simulink model "Electric_Vehicle_Dynamic"  (R2019a)
settings: Solver=VariableStepAuto  StartTime=0.0  StopTime=10.0  RelTol=1e-3
settings Model: Creator=dağlar  LastModifiedBy=dağlar

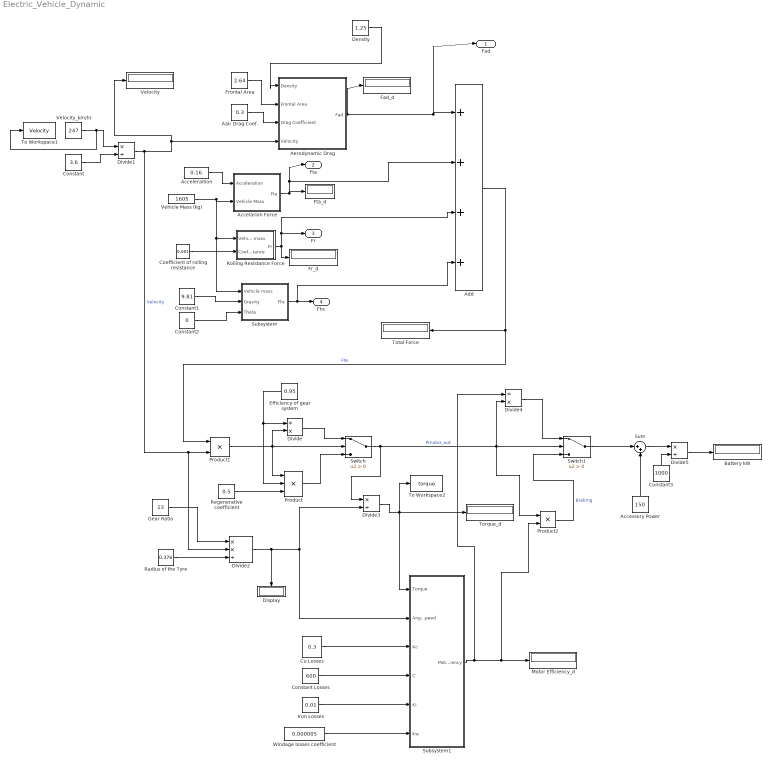
== system Electric_Vehicle_Dynamic ==
  Aair Drag Coef. : Constant  Value=0.3
  Accelarion Force : Subsystem
  Acceleraition : Constant  Value=0.16
  Accessory Power : Constant  Value=150
  Add : Sum  Inputs=++++
  "Aerodynamic Drag " : Subsystem
  Battery kW : Display
  Coefficient of rolling resistance : Constant  Value=0.001
  Constant : Constant  Value=3.6
  Constant Losses : Constant  Value=600
  Constant1 : Constant  Value=9.81
  Constant2 : Constant  Value=0
  Constant3 : Constant  Value=1000
  Cu Losses : Constant  Value=0.3
  Density : Constant  Value=1.25
  Display : Display
  Divide : Product  Inputs=/*
  Divide1 : Product  Inputs=*/
  Divide2 : Product  Inputs=**/
  Divide3 : Product  Inputs=*/
  Divide4 : Product  Inputs=/*
  Divide5 : Product  Inputs=*/
  Efficiency of gear system : Constant  Value=0.95
  "Fad_d " : Display
  Fr_d : Display
  Frontal Area : Constant  Value=2.64
  Fta_d : Display
  Gear Ratio : Constant  Value=13
  Iron Losses : Constant  Value=0.01
  Motor Efficiency_d : Display
  Product : Product  Inputs=3
  Product1 : Product
  Product2 : Product
  Radius of the Tyre : Constant  Value=0.376
  Regenerative coefficient : Constant  Value=0.5
  Rolling Resistance Force : Subsystem
  Subsystem : Subsystem
  Subsystem1 : Subsystem
  Sum : Sum  Inputs=|++
  Switch : Switch  Criteria=u2 > Threshold
  Switch1 : Switch  Criteria=u2 > Threshold
  To Workspace1 : ToWorkspace  VariableName=Velocity  SaveFormat=Timeseries  SampleTime=-1
  To Workspace2 : ToWorkspace  VariableName=torque  SaveFormat=Timeseries  SampleTime=-1
  Torque_d : Display
  Total Force : Display
  Vehicle Mass (kg) : Constant  Value=1605
  Velocity : Display
  Velocity_km/hr : Constant  Value=247
  Windage losses coefficient : Constant  Value=0.000005
  Fad : Outport
  Fta : Outport  Port=2
  Fr : Outport  Port=3
  Fhc : Outport  Port=4
  wires:
  Regenerative coefficient/1 -> Product/3
  Divide/1 -> Switch/1
  Product/1 -> Switch/3
  Efficiency of gear system/1 -> Product/2, Divide/1
  Density/1 -> "Aerodynamic Drag "/1(Density)
  Frontal Area/1 -> "Aerodynamic Drag "/2(Frontal Area)
  Aair Drag Coef./1 -> "Aerodynamic Drag "/3(Drag Coefficient)
  "Aerodynamic Drag "/1(Fad) -> Add/1, Fad/1, "Fad_d "/1
  Velocity_km/hr/1 -> To Workspace1/1, Divide1/1
  Constant/1 -> Divide1/2
  Divide1/1 -> Divide2/2, Product1/2, "Aerodynamic Drag "/4(Velocity), Velocity/1  "Velocity"
  Acceleraition/1 -> Accelarion Force/1(Acceleration)
  Vehicle Mass (kg)/1 -> Accelarion Force/2(Vehicle Mass), Rolling Resistance Force/1(Vehicle mass), Subsystem/1(Vehicle mass)
  Accelarion Force/1(Fta) -> Add/2, Fta/1, Fta_d/1
  Coefficient of rolling resistance/1 -> Rolling Resistance Force/2(Coefficient of rolling resistance)
  Rolling Resistance Force/1(Fr) -> Fr_d/1, Add/3, Fr/1
  Constant1/1 -> Subsystem/2(Gravity)
  Subsystem/1(Fhc) -> Add/4, Fhc/1
  Constant2/1 -> Subsystem/3(Theta)
  Add/1 -> Total Force/1, Product1/1  "Fte"
  Product1/1 -> Divide/2, Product/1, Switch/2
  Gear Ratio/1 -> Divide2/1
  Radius of the Tyre/1 -> Divide2/3
  Divide2/1 -> Display/1, Subsystem1/2(Angular Speed), Divide3/2
  Switch/1 -> Product2/1, Switch1/2, Divide4/2, Divide3/1  "Pmotor_out"
  Divide3/1 -> Torque_d/1, Subsystem1/1("Torque "), To Workspace2/1
  Divide4/1 -> Switch1/1
  Subsystem1/1(Motor Efficiency) -> Divide4/1, Product2/2, Motor Efficiency_d/1
  Cu Losses/1 -> Subsystem1/3(Kc)
  Constant Losses/1 -> Subsystem1/4(C)
  Product2/1 -> Switch1/3  "Braking"
  Switch1/1 -> Sum/1
  Accessory Power/1 -> Sum/2
  Iron Losses/1 -> Subsystem1/5(Ki)
  Windage losses coefficient/1 -> Subsystem1/6(Kw)
  Sum/1 -> Divide5/1
  Constant3/1 -> Divide5/2
  Divide5/1 -> Battery kW/1

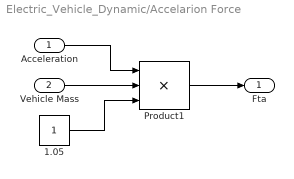
== system Electric_Vehicle_Dynamic/Accelarion Force ==
  Acceleration : Inport
  Vehicle Mass : Inport  Port=2
  "1.05 " : Constant
  Product1 : Product  Inputs=3
  Fta : Outport
  wires:
  "1.05 "/1 -> Product1/3
  Vehicle Mass/1 -> Product1/2
  Product1/1 -> Fta/1
  Acceleration/1 -> Product1/1

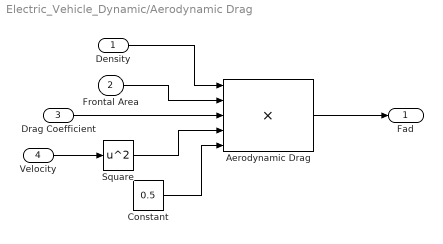
== system Electric_Vehicle_Dynamic/Aerodynamic Drag  ==
  Density : Inport
  Frontal Area : Inport  Port=2
  Drag Coefficient : Inport  Port=3
  Velocity : Inport  Port=4
  "Aerodynamic Drag " : Product  Inputs=5
  Constant : Constant  Value=0.5
  Square : Math  Operator=square  SaturateOnIntegerOverflow=on
  Fad : Outport
  wires:
  Constant/1 -> "Aerodynamic Drag "/5
  Frontal Area/1 -> "Aerodynamic Drag "/2
  Density/1 -> "Aerodynamic Drag "/1
  Square/1 -> "Aerodynamic Drag "/4
  Drag Coefficient/1 -> "Aerodynamic Drag "/3
  Velocity/1 -> Square/1
  "Aerodynamic Drag "/1 -> Fad/1

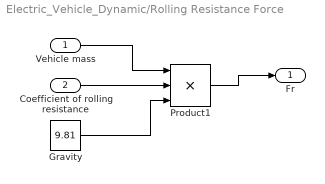
== system Electric_Vehicle_Dynamic/Rolling Resistance Force ==
  Vehicle mass : Inport
  Coefficient of rolling resistance : Inport  Port=2
  Gravity : Constant  Value=9.81
  Product1 : Product  Inputs=3
  Fr : Outport
  wires:
  Product1/1 -> Fr/1
  Gravity/1 -> Product1/3
  Coefficient of rolling resistance/1 -> Product1/2
  Vehicle mass/1 -> Product1/1

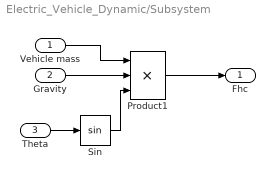
== system Electric_Vehicle_Dynamic/Subsystem ==
  Vehicle mass : Inport
  Gravity : Inport  Port=2
  Theta : Inport  Port=3
  Product1 : Product  Inputs=3
  Sin : Trigonometry
  Fhc : Outport
  wires:
  Product1/1 -> Fhc/1
  Sin/1 -> Product1/3
  Gravity/1 -> Product1/2
  Theta/1 -> Sin/1
  Vehicle mass/1 -> Product1/1

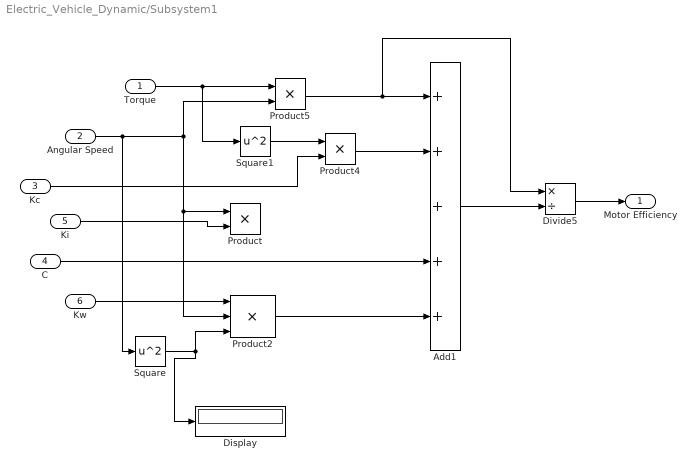
== system Electric_Vehicle_Dynamic/Subsystem1 ==
  "Torque " : Inport
  Angular Speed : Inport  Port=2
  Kc : Inport  Port=3
  C : Inport  Port=4
  Ki : Inport  Port=5
  Kw : Inport  Port=6
  Add1 : Sum  Inputs=+++++
  Display : Display
  Divide5 : Product  Inputs=*/
  Product : Product
  Product2 : Product  Inputs=3
  Product4 : Product
  Product5 : Product
  Square : Math  Operator=square  SaturateOnIntegerOverflow=on
  Square1 : Math  Operator=square  SaturateOnIntegerOverflow=on
  Motor Efficiency : Outport
  wires:
  Square1/1 -> Product4/1
  Product5/1 -> Divide5/1, Add1/1
  Angular Speed/1 -> Square/1, Product5/2, Product/1, Product2/2
  Product4/1 -> Add1/2
  Kc/1 -> Product4/2
  "Torque "/1 -> Square1/1, Product5/1
  Square/1 -> Display/1, Product2/3
  Add1/1 -> Divide5/2
  Divide5/1 -> Motor Efficiency/1
  Product2/1 -> Add1/5
  C/1 -> Add1/4
  Ki/1 -> Product/2
  Kw/1 -> Product2/1
